simulink model "dampedpendulum_differential"  (R2014a)
settings: Solver=ode3  StartTime=0.0  StopTime=50  FixedStep=1e-3  RelTol=1e-3
values from neighbouring files (symbols this model uses):
  c = 0.15    [Task4.m]
  g = 9.81    [Task4.m]
  l = 2.5    [Task4.m]
  m = 0.75    [Task4.m]
settings Model: Creator=Eduardo  LastModifiedBy=Eduardo

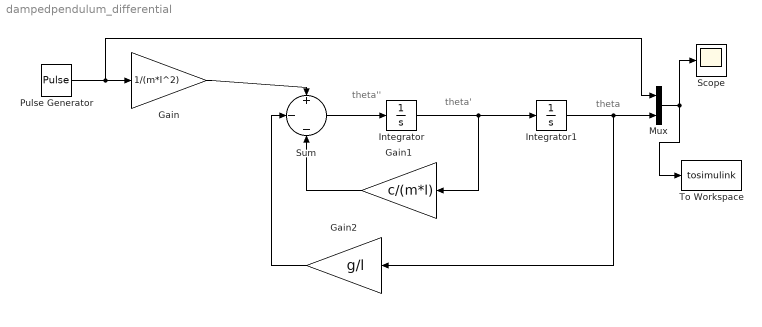
== system dampedpendulum_differential ==
  note: theta
  note: theta'
  note: theta''
  Gain : Gain  Gain=1/(m*l^2)
  Gain1 : Gain  Gain=c/(m*l)
  Gain2 : Gain  Gain=g/l
  Integrator : Integrator
  Integrator1 : Integrator
  Mux : Mux  Inputs=2
  Pulse Generator : DiscretePulseGenerator  PulseType=Time based  Amplitude=200  Period=100  PulseWidth=0.1
  Scope : Scope
  Sum : Sum  Inputs=+|-|-
  To Workspace : ToWorkspace  VariableName=tosimulink  SaveFormat=Timeseries  SampleTime=-1
  wires:
  Pulse Generator/1 -> Mux/1, Gain/1
  Gain/1 -> Sum/1
  Sum/1 -> Integrator/1
  Integrator/1 -> Integrator1/1, Gain1/1
  Gain1/1 -> Sum/3
  Gain2/1 -> Sum/2
  Mux/1 -> To Workspace/1, Scope/1
  Integrator1/1 -> Gain2/1, Mux/2
